simulink model "Ideal"  (R2025b)
settings: Solver=VariableStepAuto  StartTime=0.0  StopTime=4.608  RelTol=1e-3
values from neighbouring files (symbols this model uses):
  a1 = a(1)    [init.m]
  a2 = a(2)    [init.m]
  a3 = a(3)    [init.m]
  a4 = a(4)    [init.m]
  Ain = 1.8    [init.m]
  b1 = b(1)    [init.m]
  c1 = c(1)    [init.m]
  c2 = c(2)    [init.m]
  c3 = c(3)    [init.m]
  c4 = c(4)    [init.m]
  fin = 250    [init.m]
  fir_coefficients = firpm(MaxTaps-1, F, A, W)    [fir_coeff.m]
  fs = 128e3    (= 128000)    [init.m]
  g1 = g(1)    [init.m]
  g2 = g(2)    [init.m]
  Gj = 1e5    (= 100000)    [init.m]
  h = h / max(h)    [cic_comp_coeff_calc.m]    (also in gain_calculate.m = tf.k * evalRP(tf.zeros,z) ./ evalRP(tf.poles,z))
  halfband_coeff = firhalfband(N, kaiser(N+1, beta))    [fir_halfband_coeff.m]
  scale = 1.6    [init.m]
libraries: dsphdlfiltering2 x4, dspfdesign x1
settings Model: Creator=Rudra Thakar  LastModifiedBy=sohom

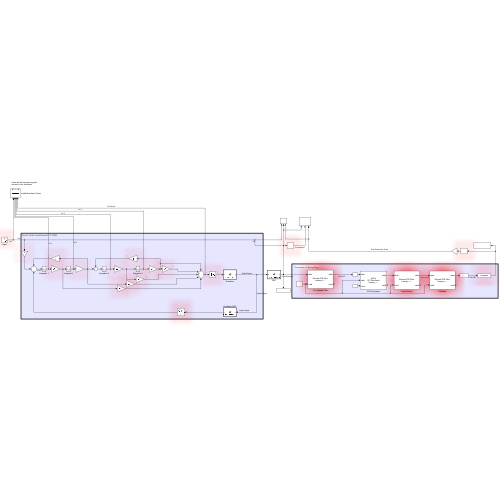
[thumbnail: Simulink's stored preview of the top-level diagram]
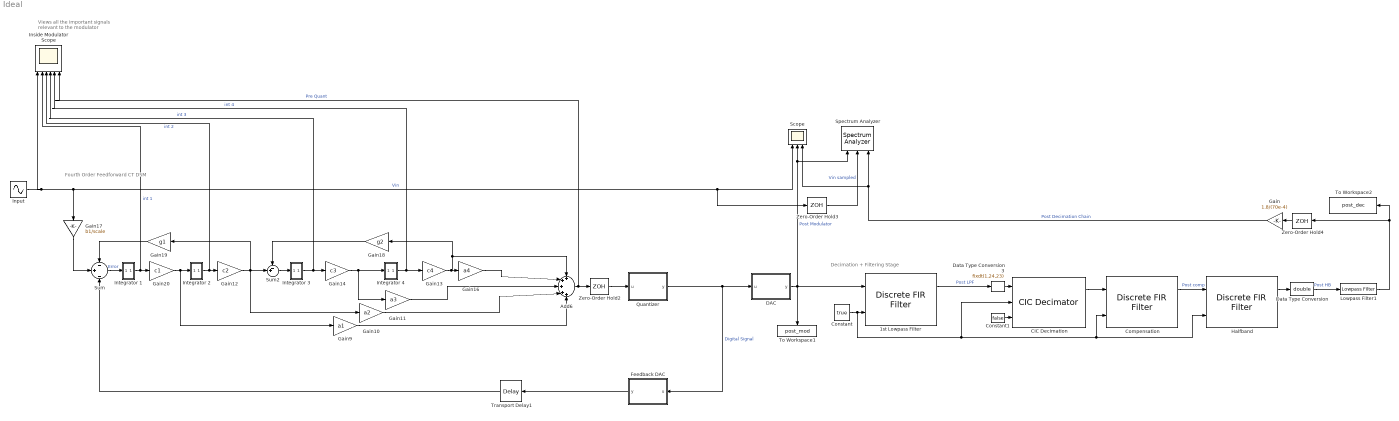
== system Ideal ==
  note: Decimation + Filtering Stage
  note: Views all the important signals
      | relevant to the modulator
  note: Fourth Order Feedforward CT DSM
  1st Lowpass Filter : dsphdlfiltering2/Discrete FIR Filter  NumeratorSource=Property  Numerator=[fir_coefficients]  NumeratorPrototype=[]  FilterStructure=Direct form systolic  SerializationOption=Minimum number of cycles between valid input samples  NumCycles=2  NumberOfMultipliers=2  SimulateUsing=Code generation  roundingMode=Floor  overflowMode=off  CoefficientsDataTypeStr=Inherit: Same word length as input  ResetInputPort=off  HDLGlobalReset=off  CoeffMultiplier=Multiplier  UseMultForPow2Coeff=on  FrameInputSymmOptim=on
  Add6 : Sum  Inputs=+++++
  CIC Decimation : dsphdlfiltering2/CIC Decimator  DecimationSource=Property  DecimationFactor=32  MaxDecimationFactor=2  DifferentialDelay=1  NumSections=5  GainCorrection=on  SimulateUsing=Code generation  OutputDataType=Full precision  OutputWordLength=16  ResetInputPort=on  HDLGlobalReset=off
  Compensation : dsphdlfiltering2/Discrete FIR Filter  NumeratorSource=Property  Numerator=[h]  NumeratorPrototype=[]  FilterStructure=Direct form systolic  SerializationOption=Minimum number of cycles between valid input samples  NumCycles=2  NumberOfMultipliers=2  SimulateUsing=Code generation  roundingMode=Floor  overflowMode=off  CoefficientsDataTypeStr=Inherit: Same word length as input  ResetInputPort=off  HDLGlobalReset=off  CoeffMultiplier=Multiplier  UseMultForPow2Coeff=on  FrameInputSymmOptim=on
  Constant : Constant  Value=true
  Constant1 : Constant  Value=false
  DAC : MATLAB Function  TreatAsAtomicUnit=on
  Data Type Conversion : DataTypeConversion  OutDataTypeStr=double  RndMeth=Nearest  SaturateOnIntegerOverflow=off
  Data Type Conversion3 : DataTypeConversion  OutDataTypeStr=fixdt(1,24,23)  RndMeth=Nearest  SaturateOnIntegerOverflow=off
  Feedback DAC : MATLAB Function  TreatAsAtomicUnit=on
  Gain : Gain  Gain=1.8/(70e-4)
  Gain10 : Gain  Gain=a2
  Gain11 : Gain  Gain=a3
  Gain12 : Gain  Gain=c2
  Gain13 : Gain  Gain=c4
  Gain14 : Gain  Gain=c3
  Gain16 : Gain  Gain=a4
  Gain17 : Gain  Gain=b1/scale
  Gain18 : Gain  Gain=g2
  Gain19 : Gain  Gain=g1
  Gain20 : Gain  Gain=c1
  Gain9 : Gain  Gain=a1
  Halfband : dsphdlfiltering2/Discrete FIR Filter  NumeratorSource=Property  Numerator=[halfband_coeff]  NumeratorPrototype=[]  FilterStructure=Direct form systolic  SerializationOption=Minimum number of cycles between valid input samples  NumCycles=2  NumberOfMultipliers=2  SimulateUsing=Code generation  roundingMode=Floor  overflowMode=off  CoefficientsDataTypeStr=Inherit: Same word length as input  ResetInputPort=off  HDLGlobalReset=off  CoeffMultiplier=Multiplier  UseMultForPow2Coeff=on  FrameInputSymmOptim=on
  Input : Sin  Amplitude=Ain  Frequency=2*pi*fin
  Inside Modulator Scope : Scope  NumInputPorts=6
      settings: ActiveDisplayYMinimum=-2.3793429624645488  ActiveDisplayYMaximum=2.2399294898040543  DataLoggingVariableName=ScopeData2
  Integrator 1 : Subsystem
  Integrator 2 : Subsystem
  Integrator 3 : Subsystem
  Integrator 4 : Subsystem
  Lowpass Filter1 : dspfdesign/Lowpass Filter  FilterType=FIR  DesignForMinimumOrder=on  FilterOrder=50  PassbandFrequency=1000  StopbandFrequency=2000  PassbandRipple=0.01  StopbandAttenuation=80  SampleRateMode=Specify on dialog  SampleRate=fs  SimulateUsing=Interpreted execution  roundingMode=Floor  coeffsDataTypeStr=fixdt(1,16)
  Quantizer : MATLAB Function  TreatAsAtomicUnit=on
  Scope : Scope  NumInputPorts=3
      settings: ActiveDisplayYMinimum=-2.2360659087505561  ActiveDisplayYMaximum=2.257708308181404
  Spectrum Analyzer : SpectrumAnalyzer  NumInputPorts=3  WindowPosition=[36.000000,-15.000000,1465.000000,844.000000,]  ScopeFrameLocation=window  SampleRate=44.1e3  PlotAsTwoSidedSpectrum=off  WindowInvariantSamplesPerUpdate=on  FrequencySpan=Start and stop frequencies  StartFrequency=20  StopFrequency=20e3  YLimits=[NaN NaN]  ShowLegend=on  SelectedToolstripTab=spectrumAnalyzerToolstrip.measurementsTab
  Sum : Sum  Inputs=-|+|-
  Sum2 : Sum  Inputs=-+|
  To Workspace1 : ToWorkspace  VariableName=post_mod  SaveFormat=Timeseries  SampleTime=-1
  To Workspace2 : ToWorkspace  VariableName=post_dec  SaveFormat=Timeseries  SampleTime=-1
  Transport Delay1 : TransportDelay  DelayTime=0.1/fs
  Zero-Order Hold2 : ZeroOrderHold  SampleTime=1/fs
  Zero-Order Hold3 : ZeroOrderHold  SampleTime=1/fs
  Zero-Order Hold4 : ZeroOrderHold  SampleTime=1/fs
  wires:
  Sum/1 -> Integrator 1/1(In1)  "Error"
  Zero-Order Hold2/1 -> Quantizer/1(u)
  Quantizer/1(y) -> DAC/1(u), Feedback DAC/1(u)  "Digital Signal"
  Integrator 2/1(Out1) -> Inside Modulator Scope/3, Gain12/1  "int 2"
  Integrator 4/1(Out1) -> Inside Modulator Scope/5, Gain13/1  "int 4"
  Gain16/1 -> Add6/2
  Gain11/1 -> Add6/3
  Gain10/1 -> Add6/4
  Add6/1 -> Inside Modulator Scope/6, Zero-Order Hold2/1  "Pre Quant"
  Zero-Order Hold3/1 -> Spectrum Analyzer/2  "Vin sampled"
  Gain17/1 -> Sum/2
  Integrator 1/1(Out1) -> Gain20/1, Inside Modulator Scope/2  "int 1"
  Sum2/1 -> Integrator 3/1(In1)
  Integrator 3/1(Out1) -> Gain14/1, Inside Modulator Scope/4  "int 3"
  Transport Delay1/1 -> Sum/3
  Gain18/1 -> Sum2/1
  Gain19/1 -> Sum/1
  Gain20/1 -> Integrator 2/1(In1), Gain9/1
  Gain12/1 -> Gain19/1, Sum2/2, Gain10/1
  Gain14/1 -> Integrator 4/1(In1), Gain11/1
  Gain13/1 -> Gain18/1, Add6/1, Gain16/1
  Input/1 -> Gain17/1, Scope/1, Zero-Order Hold3/1, Inside Modulator Scope/1  "Vin"
  Feedback DAC/1(y) -> Transport Delay1/1
  DAC/1(y) -> 1st Lowpass Filter/1, To Workspace1/1, Spectrum Analyzer/1, Scope/2  "Post Modulator"
  Constant/1 -> CIC Decimation/2, Halfband/2, Compensation/2, 1st Lowpass Filter/2
  Compensation/1 -> Halfband/1  "Post comp"
  Gain9/1 -> Add6/5
  1st Lowpass Filter/1 -> Data Type Conversion3/1  "Post LPF"
  Lowpass Filter1/1 -> Zero-Order Hold4/1, To Workspace2/1
  Data Type Conversion/1 -> Lowpass Filter1/1  "Post HB"
  Halfband/1 -> Data Type Conversion/1
  CIC Decimation/1 -> Compensation/1
  Data Type Conversion3/1 -> CIC Decimation/1
  Constant1/1 -> CIC Decimation/3
  Zero-Order Hold4/1 -> Gain/1
  Gain/1 -> Scope/3, Spectrum Analyzer/3  "Post Decimation Chain"

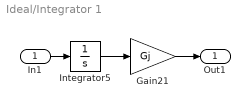
== system Ideal/Integrator 1 ==
  In1 : Inport
  Gain21 : Gain  Gain=Gj
  Integrator5 : Integrator
  Out1 : Outport
  wires:
  Gain21/1 -> Out1/1
  Integrator5/1 -> Gain21/1
  In1/1 -> Integrator5/1

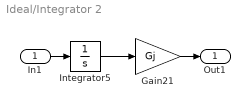
== system Ideal/Integrator 2 ==
  In1 : Inport
  Gain21 : Gain  Gain=Gj
  Integrator5 : Integrator
  Out1 : Outport
  wires:
  Gain21/1 -> Out1/1
  Integrator5/1 -> Gain21/1
  In1/1 -> Integrator5/1

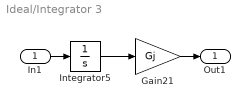
== system Ideal/Integrator 3 ==
  In1 : Inport
  Gain21 : Gain  Gain=Gj
  Integrator5 : Integrator
  Out1 : Outport
  wires:
  Gain21/1 -> Out1/1
  Integrator5/1 -> Gain21/1
  In1/1 -> Integrator5/1

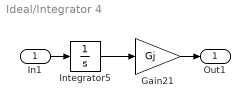
== system Ideal/Integrator 4 ==
  In1 : Inport
  Gain21 : Gain  Gain=Gj
  Integrator5 : Integrator
  Out1 : Outport
  wires:
  Gain21/1 -> Out1/1
  Integrator5/1 -> Gain21/1
  In1/1 -> Integrator5/1

== matlab function Ideal/Quantizer ==
  data: u input; y output
function y = ct_quantizer(u)
% CT DSM Quantizer with Thermometer Code Output
% Insert this as a MATLAB Function block in Simulink
%
% PARAMETERS (modify these at the top)
% =========================================================================
N_LEVELS = 16;           % Number of quantization levels (1-bit = 2 levels)
INPUT_MIN = -1.8;       % Minimum input range
INPUT_MAX = 1.8;        % Maximum input range
% =========================================================================

% Validate parameters
assert(N_LEVELS >= 2, 'N_LEVELS must be at least 2');
assert(INPUT_MAX > INPUT_MIN, 'INPUT_MAX must be greater than INPUT_MIN');

% Input saturation (clip to range)
u_clipped = max(INPUT_MIN, min(INPUT_MAX, u));

% Mid-tread quantizer: zero is a quantization level
% For N levels, we have (N-1) thresholds
if N_LEVELS == 2
    % Special case: 1-bit quantizer
    % Threshold at 0 (mid-tread)
    if u_clipped >= 0
        quant_level = 1;  % Upper level
    else
        quant_level = 0;  % Lower level
    end
else
    % Multi-bit quantizer
    % Calculate thresholds for mid-tread configuration
    % Levels are at: INPUT_MIN, ..., 0, ..., INPUT_MAX
    % Thresholds are halfway between levels
    
    % For mid-tread, ensure 0 is a level
    step = (INPUT_MAX - INPUT_MIN) / (N_LEVELS - 1);
    
    % Find which level the input corresponds to
    quant_level = round((u_clipped - INPUT_MIN) / step);
    
    % Ensure level is in valid range [0, N_LEVELS-1]
    quant_level = max(0, min(N_LEVELS - 1, quant_level));
end

% Convert to thermometer code
% Thermometer code: k ones followed by (N_LEVELS-1-k) zeros
% Example for 4 levels (3 bits):
%   Level 0 -> [0 0 0]
%   Level 1 -> [1 0 0]
%   Level 2 -> [1 1 0]
%   Level 3 -> [1 1 1]

thermometer = zeros(1, N_LEVELS - 1);
for i = 1:(N_LEVELS - 1)
    if i <= quant_level
        thermometer(i) = 1;
    end
end

% Output as column vector
y = thermometer';

% Alternative: if you want a single scalar output for 2-level case
% Uncomment the following line and comment out the thermometer code above
% if N_LEVELS == 2
%     y = 2 * quant_level - 1;  % Maps 0->-1, 1->+1
% end

end

% =========================================================================
% USAGE INSTRUCTIONS FOR SIMULINK:
% =========================================================================
% 1. Add a MATLAB Function block to your Simulink model
% 2. Double-click the block and paste this entire code
% 3. Connect the input signal (from your loop filter) to the block input
% 4. The output will be a vector of size [N_LEVELS-1 × 1] in thermometer code
%
% For 2-level (1-bit) quantizer:
%   - Input < 0  → Output = [0]   (represents -1)
%   - Input >= 0 → Output = [1]   (represents +1)
%
% For 4-level (2-bit) quantizer:
%   - Level 0 → [0 0 0]
%   - Level 1 → [1 0 0]
%   - Level 2 → [1 1 0]
%   - Level 3 → [1 1 1]
%
% NOTES:
% - To change parameters, edit N_LEVELS, INPUT_MIN, INPUT_MAX at the top
% - For single scalar output in 2-level case, use the alternative output
% - Thermometer code helps with linearity in multi-bit DACs
% =========================================================================

== matlab function Ideal/Feedback DAC ==
  data: u input; y output
function y = ct_dac_feedback(u)
% CT DSM Feedback DAC - Converts Thermometer Code to Analog Level
% Insert this as a MATLAB Function block in Simulink
% Compatible with ct_quantizer output
%
% PARAMETERS (must match quantizer settings)
% =========================================================================
N_LEVELS = 16;           % Number of quantization levels (must match quantizer)
OUTPUT_MIN = -1.8;      % Minimum output voltage/amplitude
OUTPUT_MAX = 1.8;       % Maximum output voltage/amplitude
% =========================================================================

% Validate parameters
assert(N_LEVELS >= 2, 'N_LEVELS must be at least 2');
assert(OUTPUT_MAX > OUTPUT_MIN, 'OUTPUT_MAX must be greater than OUTPUT_MIN');

% Decode thermometer code to level
% Thermometer code has (N_LEVELS - 1) bits
% Count the number of ones to get the level
if N_LEVELS == 2
    % Special case: 1-bit (single element vector)
    % u is [0] or [1]
    level = u(1);  % 0 or 1
else
    % Multi-bit: count number of ones in thermometer code
    level = sum(u);  % This gives level from 0 to (N_LEVELS-1)
end

% Convert level to analog output (mid-tread)
% Map level [0, 1, 2, ..., N_LEVELS-1] to analog range
% For mid-tread, ensure level corresponds to actual output values
if N_LEVELS == 2
    % 1-bit: simple bipolar mapping
    % Level 0 -> OUTPUT_MIN (-1.8)
    % Level 1 -> OUTPUT_MAX (+1.8)
    if level == 0
        y = OUTPUT_MIN;
    else
        y = OUTPUT_MAX;
    end
else
    % Multi-bit: linear mapping
    % Map level to output range with mid-tread alignment
    step = (OUTPUT_MAX - OUTPUT_MIN) / (N_LEVELS - 1);
    y = OUTPUT_MIN + level * step;
end

end

% =========================================================================
% USAGE INSTRUCTIONS FOR SIMULINK:
% =========================================================================
% 1. Add a MATLAB Function block after your quantizer
% 2. Double-click the block and paste this entire code
% 3. Connect quantizer output (thermometer code) to this block's input
% 4. This block's output goes to the feedback path (summed with input)
%
% SIGNAL FLOW:
%   Input → [Σ] → Loop Filter → Quantizer → Output
%            ↑                      ↓
%            └──────── DAC ─────────┘
%
% For 2-level (1-bit):
%   Thermometer [0] → Analog output = -1.8
%   Thermometer [1] → Analog output = +1.8
%
% For 4-level (2-bit):
%   Thermometer [0 0 0] → -1.8
%   Thermometer [1 0 0] → -0.6
%   Thermometer [1 1 0] → +0.6
%   Thermometer [1 1 1] → +1.8
%
% NOTES:
% - N_LEVELS, OUTPUT_MIN, OUTPUT_MAX must match quantizer parameters
% - This is an ideal DAC (no delay, noise, or mismatch)
% - For CT-DSM, this typically runs continuously (no sample/hold needed)
% - Output is continuous-time analog signal fed back to input summer
% =========================================================================

== matlab function Ideal/DAC ==
  data: u input; y output
function y = ct_dac_feedback(u)
% CT DSM Feedback DAC - Converts Thermometer Code to Analog Level
% Insert this as a MATLAB Function block in Simulink
% Compatible with ct_quantizer output
%
% PARAMETERS (must match quantizer settings)
% =========================================================================
N_LEVELS = 16;           % Number of quantization levels (must match quantizer)
OUTPUT_MIN = -1.8;      % Minimum output voltage/amplitude
OUTPUT_MAX = 1.8;       % Maximum output voltage/amplitude
% =========================================================================

% Validate parameters
assert(N_LEVELS >= 2, 'N_LEVELS must be at least 2');
assert(OUTPUT_MAX > OUTPUT_MIN, 'OUTPUT_MAX must be greater than OUTPUT_MIN');

% Decode thermometer code to level
% Thermometer code has (N_LEVELS - 1) bits
% Count the number of ones to get the level
if N_LEVELS == 2
    % Special case: 1-bit (single element vector)
    % u is [0] or [1]
    level = u(1);  % 0 or 1
else
    % Multi-bit: count number of ones in thermometer code
    level = sum(u);  % This gives level from 0 to (N_LEVELS-1)
end

% Convert level to analog output (mid-tread)
% Map level [0, 1, 2, ..., N_LEVELS-1] to analog range
% For mid-tread, ensure level corresponds to actual output values
if N_LEVELS == 2
    % 1-bit: simple bipolar mapping
    % Level 0 -> OUTPUT_MIN (-1.8)
    % Level 1 -> OUTPUT_MAX (+1.8)
    if level == 0
        y = OUTPUT_MIN;
    else
        y = OUTPUT_MAX;
    end
else
    % Multi-bit: linear mapping
    % Map level to output range with mid-tread alignment
    step = (OUTPUT_MAX - OUTPUT_MIN) / (N_LEVELS - 1);
    y = OUTPUT_MIN + level * step;
end

end

% =========================================================================
% USAGE INSTRUCTIONS FOR SIMULINK:
% =========================================================================
% 1. Add a MATLAB Function block after your quantizer
% 2. Double-click the block and paste this entire code
% 3. Connect quantizer output (thermometer code) to this block's input
% 4. This block's output goes to the feedback path (summed with input)
%
% SIGNAL FLOW:
%   Input → [Σ] → Loop Filter → Quantizer → Output
%            ↑                      ↓
%            └──────── DAC ─────────┘
%
% For 2-level (1-bit):
%   Thermometer [0] → Analog output = -1.8
%   Thermometer [1] → Analog output = +1.8
%
% For 4-level (2-bit):
%   Thermometer [0 0 0] → -1.8
%   Thermometer [1 0 0] → -0.6
%   Thermometer [1 1 0] → +0.6
%   Thermometer [1 1 1] → +1.8
%
% NOTES:
% - N_LEVELS, OUTPUT_MIN, OUTPUT_MAX must match quantizer parameters
% - This is an ideal DAC (no delay, noise, or mismatch)
% - For CT-DSM, this typically runs continuously (no sample/hold needed)
% - Output is continuous-time analog signal fed back to input summer
% =========================================================================
